simulink model "DEEE_centre_tri"  (R2026a)
settings: Solver=VariableStepDiscrete  StopTime=T_sim
values from neighbouring files (symbols this model uses):
  dt = 0.25    [params_DEEE.m]
  MTBF = 120    [params_DEEE.m]
  MTBF_B1 = 80    [params_DEEE.m]    (also in scenarios_DEEE.m = MTBF_B1_scenarios(i))
  MTBF_B2 = 120    [params_DEEE.m]
  MTBF_Mag = 200    [params_DEEE.m]
  MTBF_Opt = 60    [params_DEEE.m]
  MTTR = 4    [params_DEEE.m]
  MTTR_B1 = 6    [params_DEEE.m]
  MTTR_B2 = 4    [params_DEEE.m]
  MTTR_Mag = 3    [params_DEEE.m]
  MTTR_Opt = 2    [params_DEEE.m]
  tau_capt_GEM = 0.94    [params_DEEE.m]
undefined symbols (not defined in the file or in its folder): m, n
(part 1 of 2)
settings Model: Creator=fabri  LastModifiedBy=fabri

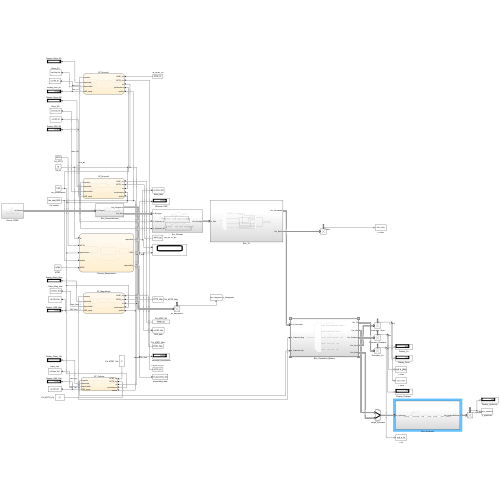
[thumbnail: Simulink's stored preview of the top-level diagram]
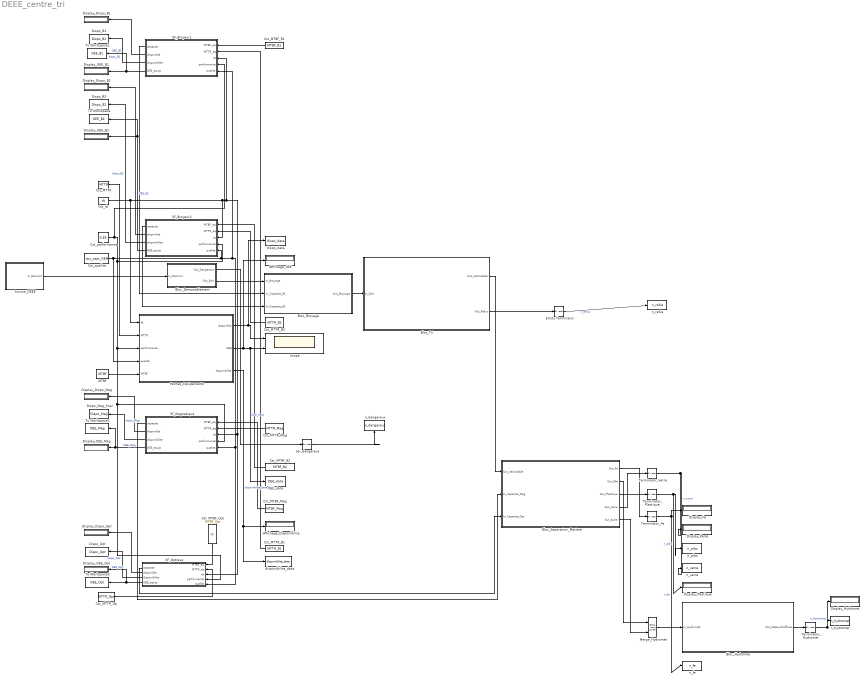
== system DEEE_centre_tri ==
  Affichage_Disponibilite : Display
  Affichage_OEE : Display
  Bloc_Broyage : Subsystem
  Bloc_Demantèlement : Subsystem
  Bloc_Hydromet : Subsystem
  Bloc_Separation_Matiere : Subsystem
  Bloc_Tri : Subsystem
  Cst_MTBF_B1 : Constant  Value=MTBF_B1
  Cst_MTBF_B2 : Constant  Value=MTBF_B2
  Cst_MTBF_Mag : Constant  Value=MTBF_Mag
  Cst_MTBF_Opt : Constant  Value=MTBF_Opt
  Cst_MTTR : Constant  Value=MTTR
  Cst_MTTR_B1 : Constant  Value=MTTR_B1
  Cst_MTTR_B2 : Constant  Value=MTTR_B2
  Cst_MTTR_Mag : Constant  Value=MTTR_Mag
  Cst_MTTR_Op : Constant  Value=MTTR_Opt
  Cst_dt : Constant  Value=dt
  Cst_performance : Constant  Value=0.85
  Cst_qualite : Constant  Value=tau_capt_GEM
  Display_Dispo_B1 : Display
  Display_Dispo_B2 : Display
  Display_Dispo_Mag : Display
  Display_Dispo_Opt : Display
  Display_Fe : Display
  Display_Hydromet : Display
  Display_OEE_B1 : Display
  Display_OEE_B2 : Display
  Display_OEE_Mag : Display
  Display_OEE_Opt : Display
  Display_Perre : Display
  Display_Plastique : Display
  Dispo_B1 : ToWorkspace  VariableName=Dispo_B1  SaveFormat=Timeseries  SampleTime=-1
  Dispo_B2 : ToWorkspace  VariableName=Dispo_B2  SaveFormat=Timeseries  SampleTime=-1
  Dispo_Mag_final : ToWorkspace  VariableName=Dispo_Mag  SaveFormat=Timeseries  SampleTime=-1
  Dispo_Opt : ToWorkspace  VariableName=Dispo_Opt  SaveFormat=Timeseries  SampleTime=-1
  Entity Terminator : EntityTerminator  InputPortMessageModes=m  NumberEntitiesArrived=on
      settings: OutputPortMap=o0
  MTBF : Constant  Value=MTBF
  Merge_Hydromet : EntityInputSwitch  InputPortMessageModes=m,m  OutputPortMessageModes=m
  OEE_data : ToWorkspace  VariableName=OEE_data  SaveFormat=Timeseries  SampleTime=-1
  Pannes_Equipements : Stateflow chart  TreatAsAtomicUnit=on
  SF_Broyeur1 : Stateflow chart  TreatAsAtomicUnit=on
  SF_Broyeur2 : Stateflow chart  TreatAsAtomicUnit=on
  SF_Magnetique : Stateflow chart  TreatAsAtomicUnit=on
  SF_Optique : Stateflow chart  TreatAsAtomicUnit=on
  Scope : Scope  NumInputPorts=2
      settings: ActiveDisplayYMinimum=-0.22946896582031268  ActiveDisplayYMaximum=1.3658829873046878
  Source_DEEE : Subsystem
  Terminator_Fe : EntityTerminator  InputPortMessageModes=m  NumberEntitiesArrived=on
      settings: OutputPortMap=o0
  Terminator_Hydromet : EntityTerminator  InputPortMessageModes=m  NumberEntitiesArrived=on
      settings: OutputPortMap=o0
  Terminator_Plastique : EntityTerminator  InputPortMessageModes=m  NumberEntitiesArrived=on
      settings: OutputPortMap=o0
  Terminator_Verre : EntityTerminator  InputPortMessageModes=m  NumberEntitiesArrived=on
      settings: OutputPortMap=o0
  To Workspace : ToWorkspace  VariableName=OEE_B2  SaveFormat=Timeseries  SampleTime=-1
  To Workspace1 : ToWorkspace  VariableName=OEE_B1  SaveFormat=Timeseries  SampleTime=-1
  To Workspace2 : ToWorkspace  VariableName=OEE_Mag  SaveFormat=Timeseries  SampleTime=-1
  To Workspace3 : ToWorkspace  VariableName=OEE_Opt  SaveFormat=Timeseries  SampleTime=-1
  dispo_data : ToWorkspace  VariableName=dispo_data  SaveFormat=Timeseries  SampleTime=-1
  disponibilite_data : ToWorkspace  VariableName=disponibilite_data  SaveFormat=Timeseries  SampleTime=-1
      settings: Save2DSignal=2-D array (concatenate along first dimension)
  n_dangereux : ToWorkspace  VariableName=n_dangereux  SaveFormat=Timeseries  SampleTime=-1
  n_fe : ToWorkspace  VariableName=n_fe  SaveFormat=Timeseries  SampleTime=-1
      settings: Save2DSignal=2-D array (concatenate along first dimension)
  n_hydromet : ToWorkspace  VariableName=n_hydromet  SaveFormat=Timeseries  SampleTime=-1
  n_plas : ToWorkspace  VariableName=n_plas  SaveFormat=Timeseries  SampleTime=-1
      settings: Save2DSignal=2-D array (concatenate along first dimension)
  n_refus : ToWorkspace  VariableName=n_refus  SaveFormat=Timeseries  SampleTime=-1
  n_verre : ToWorkspace  VariableName=n_verre  SaveFormat=Timeseries  SampleTime=-1
  ter_dangereux : EntityTerminator  InputPortMessageModes=m  NumberEntitiesArrived=on
      settings: OutputPortMap=o0
  wires:
  Source_DEEE/1(In_Demont) -> Bloc_Demantèlement/1(In_Demont)
  Cst_MTTR_Mag/1 -> SF_Magnetique/2(MTTR_eq)
  MTBF/1 -> Pannes_Equipements/5(MTBF)
  SF_Magnetique/3(disponibilite) -> Dispo_Mag_final/1  "dispo_Mag"
  Cst_qualite/1 -> SF_Magnetique/5(qualite), SF_Optique/5(qualite), SF_Broyeur1/5(qualite), SF_Broyeur2/5(qualite), Pannes_Equipements/4(qualite)
  Cst_performance/1 -> SF_Optique/4(performance), SF_Magnetique/4(performance), Pannes_Equipements/3(performance), SF_Broyeur2/4(performance), SF_Broyeur1/4(performance)
  Cst_dt/1 -> SF_Magnetique/3(dt), SF_Optique/3(dt), SF_Broyeur1/3(dt), SF_Broyeur2/3(dt), Pannes_Equipements/1(dt)
  Cst_MTTR/1 -> Pannes_Equipements/2(MTTR)
  Cst_MTBF_Opt/1 -> SF_Optique/1(MTBF_eq)
  Cst_MTBF_Mag/1 -> SF_Magnetique/1(MTBF_eq)
  Cst_MTTR_Op/1 -> SF_Optique/2(MTTR_eq)
  Cst_MTTR_B1/1 -> SF_Broyeur1/2(MTTR_eq)
  Cst_MTBF_B1/1 -> SF_Broyeur1/1(MTBF_eq)
  SF_Broyeur1/4(OEE_equip) -> To Workspace1/1, Display_OEE_B1/1  "OEE_B1"
  SF_Broyeur1/3(disponibilite) -> Dispo_B1/1  "dispo_B1"
  Pannes_Equipements/1(disponible) -> Scope/1, dispo_data/1
  SF_Broyeur1/2(disponible) -> Display_Dispo_B1/1
  SF_Broyeur1/1(capacite) -> Bloc_Broyage/2(In_Capacite_B1)
  SF_Broyeur2/4(OEE_equip) -> To Workspace/1, Display_OEE_B2/1  "OEE_B2"
  Cst_MTTR_B2/1 -> SF_Broyeur2/2(MTTR_eq)
  SF_Broyeur2/3(disponibilite) -> Dispo_B2/1  "dispo_B2"
  SF_Broyeur2/2(disponible) -> Display_Dispo_B2/1
  SF_Broyeur2/1(capacite) -> Bloc_Broyage/3(In_Capacite_B2)
  SF_Magnetique/4(OEE_equip) -> To Workspace2/1, Display_OEE_Mag/1  "OEE_Mag"
  Terminator_Fe/1 -> Display_Fe/1, n_fe/1  "n_fe"
  SF_Magnetique/2(disponible) -> Display_Dispo_Mag/1
  Cst_MTBF_B2/1 -> SF_Broyeur2/1(MTBF_eq)
  SF_Magnetique/1(capacite) -> Bloc_Separation_Matiere/2(In_Capacite_Mag)
  SF_Optique/4(OEE_equip) -> To Workspace3/1, Display_OEE_Opt/1  "OEE_Opt"
  SF_Optique/3(disponibilite) -> Dispo_Opt/1  "dispo_Opt"
  Bloc_Separation_Matiere/2(Out_Nfe) -> Merge_Hydromet/1
  SF_Optique/2(disponible) -> Display_Dispo_Opt/1
  Terminator_Hydromet/1 -> n_hydromet/1, Display_Hydromet/1  "n_hydromet"
  SF_Optique/1(capacite) -> Bloc_Separation_Matiere/3(In_Capacite_Opt)
  Pannes_Equipements/2(OEE) -> OEE_data/1, Scope/2, Affichage_OEE/1  "OEE_data"
  Bloc_Demantèlement/1(Out_Dangereux) -> ter_dangereux/1
  Bloc_Demantèlement/2(Out_Sain) -> Bloc_Broyage/1(In_Broyage)
  Pannes_Equipements/3(disponibilite) -> Affichage_Disponibilite/1, disponibilite_data/1  "disponibilite_data"
  Bloc_Broyage/1(Out_Broyage) -> Bloc_Tri/1(In_Sain)
  ter_dangereux/1 -> n_dangereux/1
  Bloc_Tri/1(Out_Valorisable) -> Bloc_Separation_Matiere/1(Out_Valorisable)
  Bloc_Tri/2(Out_Refus) -> Entity Terminator/1
  Entity Terminator/1 -> n_refus/1  "n_refus"
  Bloc_Separation_Matiere/5(Out_Autre) -> Merge_Hydromet/2
  Bloc_Separation_Matiere/1(Out_Fe) -> Terminator_Fe/1
  Bloc_Separation_Matiere/3(Out_Plastique) -> Terminator_Plastique/1
  Bloc_Hydromet/1(Out_MetauxRaffines) -> Terminator_Hydromet/1
  Bloc_Separation_Matiere/4(Out_Verre) -> Terminator_Verre/1
  Terminator_Verre/1 -> n_verre/1, Display_Perre/1  "n_verre"
  Terminator_Plastique/1 -> n_plas/1, Display_Plastique/1  "n_plas"
  Merge_Hydromet/1 -> Bloc_Hydromet/1(In_Hydromet)

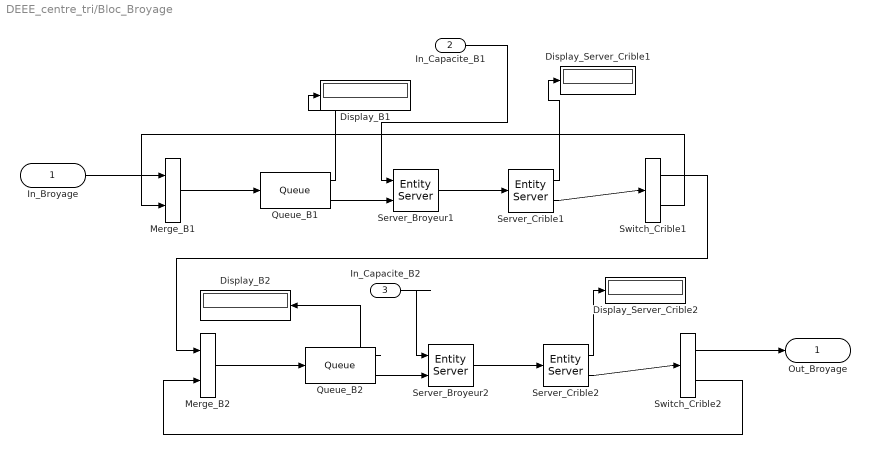
== system DEEE_centre_tri/Bloc_Broyage ==
  In_Broyage : Inport
  In_Capacite_B1 : Inport  Port=2
  In_Capacite_B2 : Inport  Port=3
  Display_B1 : Display
  Display_B2 : Display
  Display_Server_Crible1 : Display
  Display_Server_Crible2 : Display
  Merge_B1 : EntityInputSwitch  InputPortMessageModes=m,m  OutputPortMessageModes=m  SwitchingCriterion=Equiprobable
  Merge_B2 : EntityInputSwitch  InputPortMessageModes=m,m  OutputPortMessageModes=m  SwitchingCriterion=Equiprobable
  Queue_B1 : Queue  InputPortMessageModes=m  OutputPortMessageModes=n,m  Capacity=inf  NumberEntitiesInBlock=on
      settings: OutputPortMap=o1,o5
  Queue_B2 : Queue  InputPortMessageModes=m  OutputPortMessageModes=n,m  Capacity=inf  NumberEntitiesInBlock=on
      settings: OutputPortMap=o1,o5
  Server_Broyeur1 : EntityServer  InputPortMessageModes=n,m  OutputPortMessageModes=m  Capacity=10  ServiceTimeSource=Signal port  ServiceTimeAttributeName=tps_service  EntryAction=|
      | % =SÉCURITÉ DES ATTRIBUTS=
      | entity.grain_route       = 1;
      | entity.route_depollution = 2;
      | entity.valorisable       = 1;
      | cat = entity.categorie;
      | if isempty(cat) || ~isscalar(cat) || cat < 1 || cat > 4
      |     cat = 1;
      |     entity.categorie = 1;
      | end
      | 
      | % =BROYAGE PRIMAIRE (marteaux)=
      | r1_moy = [6.0, 7.0, 5.0, 8.0];
      | r1 = r1_moy(cat) * (1 + 0.15*(2*rand()-1));
      | r1 = max(r1, 1.0);
      | 
      | % Granulométrie d'entrée
      | if entity.granulometrie <= 0
      |     d50_init = [200, 100, 150, 120];
      |     entity.granulometrie = d50_init(cat) * (1 + 0.2*(2*rand()-1));
      | end
      | entity.granulometrie = entity.granulometrie / r1;
      | entity.granulometrie = max(entity.granulometrie, 0.5);
      | 
      | % Compteur de passages
      | entity.nb_passages = entity.nb_passages + 1;
      | 
      | % Temps de service
      | entity.tps_service = max(entity.masse / 6.0, 0.001);
      | 
      | % Rendement matière
      | entity.masse = max(entity.masse * 0.95, 0.0001);
      | % Énergie broyage primaire
      | energie_spec_B1 = 15.0;   % kWh/tonne
      | entity.energie_broyage = entity.energie_broyage + ...
      |     entity.masse * 1000 * energie_spec_B1 / 1000;  % kWh
      settings: InputPortMap=u0,u2
  Server_Broyeur2 : EntityServer  InputPortMessageModes=n,m  OutputPortMessageModes=m  Capacity=10  ServiceTimeSource=Signal port  ServiceTimeAttributeName=tps_service  EntryAction=|
      | % = SÉCURITÉ ATTRIBUTS =
      | entity.grain_route       = 1;
      | entity.route_depollution = 2;
      | entity.valorisable       = 1;
      | cat = entity.categorie;
      | if isempty(cat) || ~isscalar(cat) || cat < 1 || cat > 4
      |     cat = 1;
      |     entity.categorie = 1;
      | end
      | 
      | % = BROYAGE SECONDAIRE (boulets) =
      | r2_moy = [8.0, 10.0, 7.0, 9.0];
      | r2 = r2_moy(cat) * (1 + 0.15*(2*rand()-1));
      | r2 = max(r2, 1.0);
      | 
      | entity.granulometrie = entity.granulometrie / r2;
      | entity.granulometrie = max(entity.granulometrie, 0.1);
      | 
      | % Compteur de passages
      | entity.nb_passages = entity.nb_passages + 1;
      | 
      | % Temps de service
      | entity.tps_service = max(entity.masse / 3.0, 0.001);
      | 
      | % Rendement matière
      | entity.masse = max(entity.masse * 0.97, 0.0001);
      | % Énergie broyage secondaire
      | energie_spec_B2 = 25.0;   % kWh/tonne
      | entity.energie_broyage = entity.energie_broyage + ...
      |     entity.masse * 1000 * energie_spec_B2 / 1000;
      | 
      | % Énergie cribles + convoyeurs
      | energie_spec_conv = 2.0;   % kWh/tonne
      | entity.energie_broyage = entity.energie_broyage + ...
      |     entity.masse * 1000 * energie_spec_conv / 1000;
      settings: InputPortMap=u0,u2
  Server_Crible1 : EntityServer  InputPortMessageModes=m  OutputPortMessageModes=n,m  Capacity=10  ServiceTimeSource=Attribute  ServiceTimeAttributeName=tps_service  EntryAction=|  NumberEntitiesDeparted=on
      | % = SÉCURITÉ ATTRIBUTS =
      | entity.route_depollution = 2;
      | entity.valorisable       = 1;
      | if ~isscalar(entity.categorie) || entity.categorie < 1 || entity.categorie > 4
      |     entity.categorie = 1;
      | end
      | 
      | % = CRIBLAGE 1 — seuil 10mm =
      | entity.tps_service = 0.005;
      | entity.grain_route = 1;  % passant par défaut
      | 
      | if entity.nb_passages >= 3
      |     entity.grain_route = 1;  % forcer sortie après 3 passages
      | elseif entity.granulometrie > 10.0
      |     entity.grain_route = 2;  % refus → recirculation B1
      | end
      settings: OutputPortMap=o0,o9
  Server_Crible2 : EntityServer  InputPortMessageModes=m  OutputPortMessageModes=n,m  Capacity=10  ServiceTimeSource=Attribute  ServiceTimeAttributeName=tps_service  EntryAction=|  NumberEntitiesDeparted=on
      | % = SÉCURITÉ ATTRIBUTS =
      | entity.route_depollution = 2;
      | entity.valorisable       = 1;
      | if ~isscalar(entity.categorie) || entity.categorie < 1 || entity.categorie > 4
      |     entity.categorie = 1;
      | end
      | 
      | % = CRIBLAGE 2 — seuil 2mm =
      | entity.tps_service = 0.005;
      | entity.grain_route = 1;  % passant par défaut
      | 
      | if entity.nb_passages >= 6
      |     entity.grain_route = 1;  % forcer la sortie après 6 passages total
      | elseif entity.granulometrie > 2.0
      |     entity.grain_route = 2;  % refus → recirculation B2
      | end
      settings: OutputPortMap=o0,o9
  Switch_Crible1 : EntityOutputSwitch  InputPortMessageModes=m  OutputPortMessageModes=m,m  SwitchingCriterion=From attribute  SwitchAttributeName=grain_route
  Switch_Crible2 : EntityOutputSwitch  InputPortMessageModes=m  OutputPortMessageModes=m,m  SwitchingCriterion=From attribute  SwitchAttributeName=grain_route
  Out_Broyage : Outport
  wires:
  Server_Crible2/2 -> Switch_Crible2/1
  Server_Crible1/2 -> Switch_Crible1/1
  Server_Broyeur2/1 -> Server_Crible2/1
  Server_Broyeur1/1 -> Server_Crible1/1
  Queue_B2/2 -> Server_Broyeur2/2
  Queue_B1/2 -> Server_Broyeur1/2
  Merge_B1/1 -> Queue_B1/1
  Merge_B2/1 -> Queue_B2/1
  Switch_Crible1/1 -> Merge_B2/1
  Switch_Crible1/2 -> Merge_B1/2
  Switch_Crible2/2 -> Merge_B2/2
  Switch_Crible2/1 -> Out_Broyage/1
  Queue_B1/1 -> Display_B1/1
  Queue_B2/1 -> Display_B2/1
  Server_Crible2/1 -> Display_Server_Crible2/1
  Server_Crible1/1 -> Display_Server_Crible1/1
  In_Broyage/1 -> Merge_B1/1
  In_Capacite_B1/1 -> Server_Broyeur1/1
  In_Capacite_B2/1 -> Server_Broyeur2/1

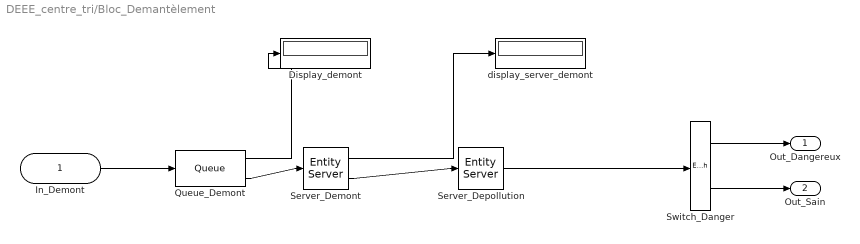
== system DEEE_centre_tri/Bloc_Demantèlement ==
  In_Demont : Inport
  Display_demont : Display
  Queue_Demont : Queue  InputPortMessageModes=m  OutputPortMessageModes=n,m  NumberEntitiesDeparted=on
      settings: OutputPortMap=o0,o5
  Server_Demont : EntityServer  InputPortMessageModes=m  OutputPortMessageModes=n,m  Capacity=20  EntryAction=|  NumberEntitiesInBlock=on
      | % Temps de démantèlement par catégorie [h]
      | % GEM=45min  PAM=15min  ECR=20min  IT=30min
      | t_demont = [0.0375, 0.0125, 0.0165, 0.0250];
      | cat = entity.categorie;
      | entity.tps_service = t_demont(cat)
      | 
      | % Granulométrie des composants après démantèlement [mm]
      | % Moyenne pondérée par composition matière
      | d50_metaux    = [150, 100,  80, 100];
      | d50_plastique = [300, 200, 250, 180];
      | d50_cartes    = [ 80,  60, 120, 150];
      | 
      | entity.granulometrie = ...
      |     (entity.masse_fe + entity.masse_nfe) / entity.masse * d50_metaux(cat) + ...
      |     entity.masse_plastique / entity.masse * d50_plastique(cat) + ...
      |     entity.masse_autre / entity.masse * d50_cartes(cat) + ...
      |     entity.masse_verre / entity.masse * 50;
      | 
      | % Variabilité ±20%
      | entity.granulometrie = entity.granulometrie * (1 + 0.20*(2*rand()-1));
      | entity.granulometrie = max(entity.granulometrie, 5);
      settings: OutputPortMap=o1,o9
  Server_Depollution : EntityServer  InputPortMessageModes=m  OutputPortMessageModes=m  Capacity=20  EntryAction=|
      | % Probabilité des substances dangereuses par catégorie
      | % GEM=15%  PAM=8%  ECR=20%  IT=12%
      | p_danger = [0.15, 0.08, 0.20, 0.12];
      | cat = entity.categorie;
      | 
      | % Détection substances dangereuses
      | if rand() < p_danger(cat)
      |     entity.dangereux = 1;
      | else
      |     entity.dangereux = 0;
      | end
      | 
      | % Masse batteries par catégorie [kg]
      | m_bat = [0.5, 0.1, 0.3, 0.2];
      | if entity.dangereux == 1
      |     entity.masse_bat = entity.masse * 1000 * m_bat(cat) / 35;
      |     entity.masse_Hg  = entity.masse * 1000 * 0.005;
      | else
      |     entity.masse_bat = 0;
      |     entity.masse_Hg  = 0;
      | end
      | 
      | % Mise à jour masse après extraction dangereuses
      | entity.masse = entity.masse - entity.masse_bat/1000;
      | entity.masse = max(entity.masse, 0.001);
      | 
      | % Temps de dépollution
      | entity.tps_service = 0.005;  % 18 secondes
      | 
      | % Routage CORRIGÉ
      | % Out_Dangereux = port 1, Out_Sain = port 2
      | if entity.dangereux == 1
      |     entity.route_depollution = 1;  % port 1 → Out_Dangereux
      | else
      |     entity.route_depollution = 2;  % port 2 → Out_Sain
      | end
  Switch_Danger : EntityOutputSwitch  InputPortMessageModes=m  OutputPortMessageModes=m,m  SwitchingCriterion=From attribute  SwitchAttributeName=route_depollution
  display_server_demont : Display
  Out_Dangereux : Outport
  Out_Sain : Outport  Port=2
  wires:
  In_Demont/1 -> Queue_Demont/1
  Queue_Demont/2 -> Server_Demont/1
  Server_Demont/2 -> Server_Depollution/1
  Server_Depollution/1 -> Switch_Danger/1
  Queue_Demont/1 -> Display_demont/1
  Server_Demont/1 -> display_server_demont/1
  Switch_Danger/2 -> Out_Sain/1
  Switch_Danger/1 -> Out_Dangereux/1

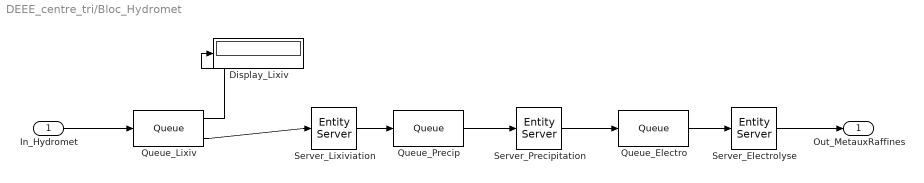
== system DEEE_centre_tri/Bloc_Hydromet ==
  In_Hydromet : Inport
  Display_Lixiv : Display
  Queue_Electro : Queue  InputPortMessageModes=m  OutputPortMessageModes=m
  Queue_Lixiv : Queue  InputPortMessageModes=m  OutputPortMessageModes=n,m  NumberEntitiesInBlock=on
      settings: OutputPortMap=o1,o5
  Queue_Precip : Queue  InputPortMessageModes=m  OutputPortMessageModes=m
  Server_Electrolyse : EntityServer  InputPortMessageModes=m  OutputPortMessageModes=m  Capacity=1  EntryAction=|
      | % Électrolyse—raffinage final
      | % Électrolyse Cu : anode impure → cathode pure 99.99%
      | % Coupellation Au/Ag : fusion + oxydation impuretés
      | 
      | % Rendements électrolyse
      | eta_electro_Cu = 0.99;
      | eta_electro_Au = 0.998;
      | eta_electro_Ag = 0.995;
      | 
      | % Masses finales raffinées [kg/g]
      | entity.masse_Cu = entity.masse_Cu * eta_electro_Cu;
      | entity.masse_Au = entity.masse_Au * eta_electro_Au;
      | entity.masse_Ag = entity.masse_Ag * eta_electro_Ag;
      | 
      | % Valeur finale après raffinage complet
      | entity.valeur_euro = entity.masse_Cu * 8.5 + ...
      |     entity.masse_Au  * 60.0 + ...
      |     entity.masse_Ag  * 0.8;
      | 
      | % Temps électrolyse—plus long pour Cu
      | % [GEM, PAM, ECR, IT]
      | t_electro = [0.15, 0.10, 0.20, 0.25];
      | cat = entity.categorie;
      | entity.tps_service = t_electro(cat);
      | % Calcul rendements globaux hydromet
      | if entity.masse_Cu_init > 0
      |     entity.rendement_Cu = entity.masse_Cu / entity.masse_Cu_init * 100;
      | else
      |     entity.rendement_Cu = 0;
      | end
      | if entity.masse_Au_init > 0
      |     entity.rendement_Au = entity.masse_Au / entity.masse_Au_init * 100;
      | else
      |     entity.rendement_Au = 0;
      | end
      | if entity.masse_Ag_init > 0
      |     entity.rendement_Ag = entity.masse_Ag / entity.masse_Ag_init * 100;
      | else
      |     entity.rendement_Ag = 0;
      | end
      | 
      | % Valeur économique finale
      | entity.valeur_euro = entity.masse_Cu * 8.5 + ...
      |     entity.masse_Au  * 60.0 + ...
      |     entity.masse_Ag  * 0.8;
      | % --- ÉNERGIE ÉLECTROLYSE ---
      | % Cu : 0.35 kWh/kg Cu récupéré
      | % Au/Ag : 0.05 kWh/g métal précieux
      | energie_Cu    = entity.masse_Cu * 1000 * 0.35;
      | energie_AuAg  = (entity.masse_Au + entity.masse_Ag) * 0.05;
      | entity.energie_electro = energie_Cu + energie_AuAg;
      | 
      | % --- ÉNERGIE TOTALE HYDROMET ---
      | entity.energie_totale = entity.energie_lixiv + ...
      |     entity.energie_precip + ...
      |     entity.energie_electro;
      | 
      | % --- EFFLUENTS FINAUX ---
      | % Traitement final — neutralisation à la chaux
      | entity.pH_effluent = 7.0 + randn() * 0.3;  % pH ≈ 7 après traitement
      | entity.conc_acide  = 0;  % acide neutralisé
      | % Énergie totale process complet
      | entity.energie_totale_process = entity.energie_broyage + ...
      |     entity.energie_tri + ...
      |     entity.energie_separation + ...
      |     entity.energie_lixiv + ...
      |     entity.energie_precip + ...
      |     entity.energie_electro;
      | %% === RÉCUPÉRATION CHALEUR ÉLECTROLYSE ===
      | 
      | % Chaleur effet Joule — 30% de l'énergie électrique dissipée
      | facteur_joule    = 0.30;
      | Q_joule_kWh      = entity.energie_electro * facteur_joule;
      | 
      | % Récupération via échangeur sur l'électrolyte chaud
      | eta_recup_electro = 0.65;   % rendement récupération électrolyse
      | Q_recup_electro   = eta_recup_electro * Q_joule_kWh;
      | 
      | % Mise à jour chaleur récupérée totale
      | entity.chaleur_recuperee = entity.chaleur_recuperee + Q_recup_electro;
      | 
      | % Énergie électrolyse nette
      | entity.energie_electro = entity.energie_electro - Q_recup_electro;
      | entity.energie_electro = max(entity.energie_electro, 0);
      | 
      | % Taux de récupération global [%]
      | energie_brute_totale = entity.energie_broyage + entity.energie_tri + ...
      |     entity.energie_separation + entity.energie_lixiv + ...
      |     entity.energie_precip + entity.energie_electro + ...
      |     entity.chaleur_recuperee;
      | 
      | if energie_brute_totale > 0
      |     entity.taux_recuperation = entity.chaleur_recuperee / ...
      |         energie_brute_totale * 100;
      | end
      | 
      | % Énergie totale nette finale
      | entity.energie_totale_process = entity.energie_broyage + ...
      |     entity.energie_tri + ...
      |     entity.energie_separation + ...
      |     entity.energie_lixiv_nette + ...
      |     entity.energie_precip + ...
      |     entity.energie_electro;
  Server_Lixiviation : EntityServer  InputPortMessageModes=m  OutputPortMessageModes=m  Capacity=1  EntryAction=|
      | %% === LIXIVIATION AVEC THERMIQUE + ENERGIE + EFFLUENTS ===
      | 
      | % --- 1. MODÉLISATION THERMIQUE ---
      | % Température initiale cuve [°C]
      | T_amb     = 20.0;   % température ambiante
      | T_cible   = 70.0;   % température opératoire cible
      | tau_chauf = 2.0;    % constante de temps chauffage [h]
      | 
      | % Montée en température (modèle du premier ordre)
      | % T(t) = T_cible - (T_cible - T_amb) * exp(-t/tau)
      | % On utilise tps_service comme proxy du temps
      | t_lixiv_base = 0.025;
      | entity.tps_service = t_lixiv_base * (entity.granulometrie / 2.0)^0.3;
      | entity.tps_service = max(entity.tps_service, 0.005);
      | entity.tps_service = min(entity.tps_service, 0.10);
      | 
      | % Température atteinte en fin de lixiviation
      | entity.temp_cuve = T_cible - (T_cible - T_amb) * ...
      |     exp(-entity.tps_service / tau_chauf);
      | 
      | % --- 2. RENDEMENTS CORRIGÉS PAR TEMPÉRATURE ---
      | % η(T) = η_ref × (1 + α × (T - T_ref))
      | T_ref  = 60.0;   % température de référence [°C]
      | alpha  = 0.005;  % coefficient température [1/°C]
      | facteur_T = 1 + alpha * (entity.temp_cuve - T_ref);
      | facteur_T = max(0.8, min(1.2, facteur_T));  % limité ±20%
      | 
      | cat = entity.categorie;
      | eta_lixiv_Cu = [0.88, 0.90, 0.85, 0.92];
      | eta_lixiv_Au = [0.80, 0.82, 0.85, 0.87];
      | eta_lixiv_Ag = [0.83, 0.85, 0.88, 0.90];
      | 
      | % Application correction thermique
      | entity.eta_lixiv_reel = eta_lixiv_Cu(cat) * facteur_T;
      | entity.masse_Cu = entity.masse_Cu * entity.eta_lixiv_reel;
      | entity.masse_Au = entity.masse_Au * eta_lixiv_Au(cat) * facteur_T;
      | entity.masse_Ag = entity.masse_Ag * eta_lixiv_Ag(cat) * facteur_T;
      | 
      | % --- 3. BILAN ÉNERGÉTIQUE LIXIVIATION ---
      | % Énergie chauffage : Q = m_cuve × Cp × ΔT / η_chauffage
      | % Simplifié : 0.8 kWh/kg de matière traitée
      | energie_spec_lixiv = 0.8;   % kWh/kg
      | entity.energie_lixiv = entity.masse * 1000 * energie_spec_lixiv;
      | 
      | % --- 4. EFFLUENTS ACIDES ---
      | % Volume effluent = 4 L/kg traité (moyenne industrielle)
      | vol_spec = [3.5, 4.0, 4.5, 5.0];   % L/kg par catégorie
      | entity.volume_effluent = entity.masse * 1000 * vol_spec(cat);
      | 
      | % pH effluent en sortie lixiviation
      | % Plus la teneur en métaux est élevée, plus le pH remonte
      | pH_base = 1.2;
      | entity.pH_effluent = pH_base + 0.5 * entity.eta_lixiv_reel;
      | 
      | % Concentration acide résiduel [mol/L]
      | entity.conc_acide = 0.5 * (1 - entity.eta_lixiv_reel);
      | %% === MODULE RÉCUPÉRATION DE CHALEUR ===
      | 
      | % Paramètres échangeur de chaleur
      | eta_echangeur = 0.75;   % rendement échangeur à plaques
      | Cp_eau        = 4.18;   % kJ/kg·°C
      | T_effluent    = entity.temp_cuve;   % température effluent sortant
      | T_reseau      = 20.0;   % température eau réseau entrant [°C]
      | T_prechauffee = T_reseau + eta_echangeur * (T_effluent - T_reseau);
      | 
      | % Masse effluent [kg] = volume [L] × densité ≈ 1 kg/L
      | masse_effluent = entity.volume_effluent;   % kg
      | 
      | % Chaleur récupérée [kWh]
      | % Q = m × Cp × ΔT / 3600 (conversion kJ → kWh)
      | Q_recuperee = masse_effluent * Cp_eau * ...
      |     (T_effluent - T_reseau) * eta_echangeur / 3600;
      | entity.chaleur_recuperee = Q_recuperee;
      | 
      | % Chaleur nécessaire SANS récupération [kWh]
      | % Q_brute = m × Cp × (T_cible - T_reseau) / 3600
      | Q_brute = masse_effluent * Cp_eau * ...
      |     (entity.temp_cuve - T_reseau) / 3600;
      | 
      | % Énergie lixiviation nette AVEC récupération
      | entity.energie_lixiv_nette = max(entity.energie_lixiv - Q_recuperee, 0);
      | 
      | % Taux de récupération [%]
      | if Q_brute > 0
      |     entity.taux_recuperation = Q_recuperee / Q_brute * 100;
      | else
      |     entity.taux_recuperation = 0;
      | end
      | 
      | % Mise à jour énergie totale avec récupération
      | entity.energie_totale_process = entity.energie_broyage + ...
      |     entity.energie_tri + ...
      |     entity.energie_separation + ...
      |     entity.energie_lixiv_nette + ...
      |     entity.energie_precip + ...
      |     entity.energie_electro;
  Server_Precipitation : EntityServer  InputPortMessageModes=m  OutputPortMessageModes=m  Capacity=1  EntryAction=|
      | % Précipitation sélective—séparation Cu/Au/Ag
      | % Étape 1 : ciment Cu (Fe + CuSO4 → FeSO4 + Cu)
      | % Étape 2 : NaOH pour précipiter Au/Ag
      | 
      | % Rendements précipitation
      | eta_precip_Cu = 0.95;
      | eta_precip_Au = 0.92;
      | eta_precip_Ag = 0.90;
      | 
      | % Masses après précipitation
      | entity.masse_Cu = entity.masse_Cu * eta_precip_Cu;
      | entity.masse_Au = entity.masse_Au * eta_precip_Au;
      | entity.masse_Ag = entity.masse_Ag * eta_precip_Ag;
      | 
      | % Temps précipitation—plus rapide que lixiviation
      | entity.tps_service = 0.075
      | 
      | % Mise à jour valeur après pertes précipitation
      | entity.valeur_euro = entity.masse_Cu * 8.5 + ...
      |     entity.masse_Au  * 60.0 + ...
      |     entity.masse_Ag  * 0.8;
      | % --- ÉNERGIE PRÉCIPITATION ---
      | energie_spec_precip = 0.1;   % kWh/kg
      | entity.energie_precip = entity.masse * 1000 * energie_spec_precip;
      | 
      | % --- EFFLUENTS PRÉCIPITATION ---
      | % Neutralisation partielle — pH remonte
      | entity.pH_effluent = entity.pH_effluent + 1.5;
      | entity.conc_acide  = entity.conc_acide * 0.3;  % 70% neutralisé
      | entity.volume_effluent = entity.volume_effluent * 0.8;  % évaporation
      | %% === RÉCUPÉRATION CHALEUR PRÉCIPITATION ===
      | 
      | % Chaleur de réaction exothermique [kWh]
      | % Cémentation Cu : ΔH ≈ -210 kJ/mol Cu
      | % Masse molaire Cu = 63.5 g/mol
      | moles_Cu = entity.masse_Cu * 1000 / 0.0635;   % moles Cu précipité
      | DH_cementation = 210;   % kJ/mol
      | Q_reaction_kJ  = moles_Cu * DH_cementation;
      | Q_reaction_kWh = Q_reaction_kJ / 3600;
      | 
      | % Récupération chaleur réaction
      | eta_recup_precip = 0.60;   % rendement récupération précipitation
      | Q_recup_precip   = eta_recup_precip * Q_reaction_kWh;
      | 
      | % Mise à jour énergie précipitation nette
      | entity.chaleur_recuperee  = entity.chaleur_recuperee + Q_recup_precip;
      | entity.energie_precip     = max(entity.energie_precip - Q_recup_precip, 0);
      | 
      | % Température effluent précipitation
      | entity.temp_cuve = 40.0 + randn() * 3.0;   % °C ≈ 40°C
  Out_MetauxRaffines : Outport
  wires:
  In_Hydromet/1 -> Queue_Lixiv/1
  Server_Precipitation/1 -> Queue_Electro/1
  Server_Lixiviation/1 -> Queue_Precip/1
  Queue_Precip/1 -> Server_Precipitation/1
  Queue_Electro/1 -> Server_Electrolyse/1
  Server_Electrolyse/1 -> Out_MetauxRaffines/1
  Queue_Lixiv/2 -> Server_Lixiviation/1
  Queue_Lixiv/1 -> Display_Lixiv/1

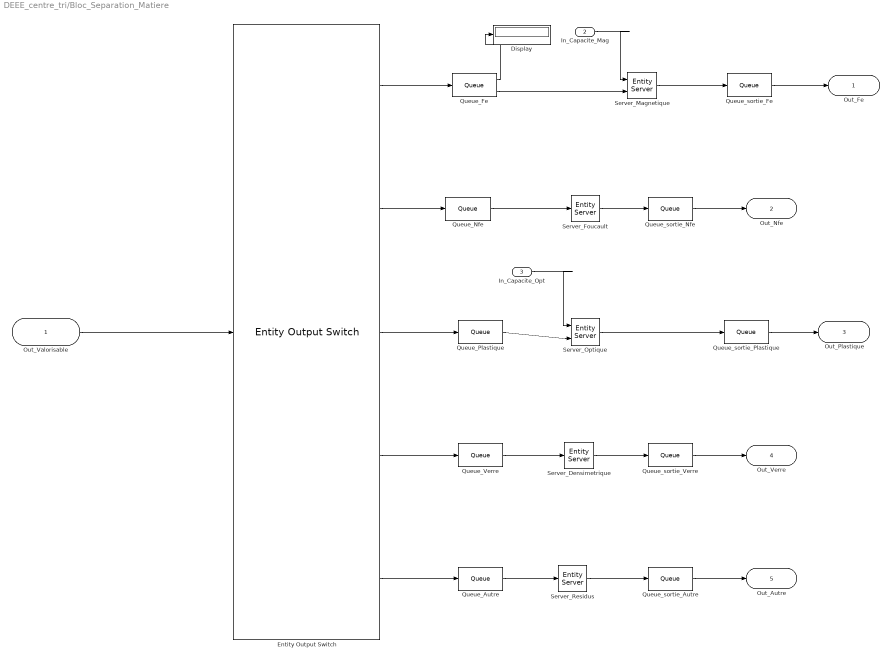
== system DEEE_centre_tri/Bloc_Separation_Matiere ==
  Out_Valorisable : Inport
  In_Capacite_Mag : Inport  Port=2
  In_Capacite_Opt : Inport  Port=3
  Display : Display
  Entity Output Switch : EntityOutputSwitch  InputPortMessageModes=m  OutputPortMessageModes=m,m,m,m,m  NumberOutputPorts=5  SwitchingCriterion=From attribute  SwitchAttributeName=fraction_dominante
      settings: OutputPortMap=o0,o1,o2,o3,o4
  Queue_Autre : Queue  InputPortMessageModes=m  OutputPortMessageModes=m
  Queue_Fe : Queue  InputPortMessageModes=m  OutputPortMessageModes=n,m  NumberEntitiesInBlock=on
      settings: OutputPortMap=o1,o5
  Queue_Nfe : Queue  InputPortMessageModes=m  OutputPortMessageModes=m
  Queue_Plastique : Queue  InputPortMessageModes=m  OutputPortMessageModes=m
  Queue_Verre : Queue  InputPortMessageModes=m  OutputPortMessageModes=m
  Queue_sortie_Autre : Queue  InputPortMessageModes=m  OutputPortMessageModes=m
  Queue_sortie_Fe : Queue  InputPortMessageModes=m  OutputPortMessageModes=m
  Queue_sortie_Nfe : Queue  InputPortMessageModes=m  OutputPortMessageModes=m
  Queue_sortie_Plastique : Queue  InputPortMessageModes=m  OutputPortMessageModes=m
  Queue_sortie_Verre : Queue  InputPortMessageModes=m  OutputPortMessageModes=m
  Server_Densimetrique : EntityServer  InputPortMessageModes=m  OutputPortMessageModes=m  Capacity=1  ServiceTimeSource=Attribute  ServiceTimeAttributeName=tps_service  EntryAction=|
      | % Rendements de séparation par procédé
      | % === SÉPARATION DENSIMÉTRIQUE — Verre ===
      | eta_densi = 0.80;
      | 
      | % Masse récupérée verre
      | entity.masse_recuperee = entity.masse_verre * eta_densi;
      | 
      | % Impuretés dans le produit verre
      | impurete_plas   = entity.masse_plastique * 0.02;
      | impurete_autre  = entity.masse_autre     * 0.02;
      | masse_sortie_Verre = entity.masse_recuperee + impurete_plas + impurete_autre;
      | 
      | % KPIs séparation densimétrique
      | if masse_sortie_Verre > 0
      |     entity.purete_Verre    = entity.masse_recuperee / masse_sortie_Verre;
      | else
      |     entity.purete_Verre    = 0;
      | end
      | entity.rendement_Verre = entity.masse_recuperee / max(entity.masse_verre, 0.0001);
      | entity.pertes_Verre    = entity.masse_verre - entity.masse_recuperee;
      | 
      | % Temps service
      | entity.tps_service = entity.masse / 2.0;
  Server_Foucault : EntityServer  InputPortMessageModes=m  OutputPortMessageModes=m  Capacity=1  ServiceTimeSource=Attribute  ServiceTimeAttributeName=tps_service  EntryAction=|
      | % Rendements de séparation par procédé
      | % === COURANTS DE FOUCAULT — Métaux non ferreux (Cu, Al) ===
      | eta_foucault = 0.85;
      | 
      | % Masse récupérée NFe
      | entity.masse_recuperee = entity.masse_nfe * eta_foucault;
      | 
      | % Impuretés dans le produit NFe
      | impurete_fe     = entity.masse_fe    * 0.02;
      | impurete_autre  = entity.masse_autre * 0.03;
      | masse_sortie_NFe = entity.masse_recuperee + impurete_fe + impurete_autre;
      | 
      | % KPIs courants de Foucault
      | if masse_sortie_NFe > 0
      |     entity.purete_NFe    = entity.masse_recuperee / masse_sortie_NFe;
      | else
      |     entity.purete_NFe    = 0;
      | end
      | entity.rendement_NFe = entity.masse_recuperee / max(entity.masse_nfe, 0.0001);
      | entity.pertes_NFe    = entity.masse_nfe - entity.masse_recuperee;
      | 
      | % Temps service
      | entity.tps_service = entity.masse / 4.0;
      | % Énergie courants de Foucault
      | energie_spec_nfe = 3.0;   % kWh/tonne
      | entity.energie_separation = entity.energie_separation + ...
      |     entity.masse * 1000 * energie_spec_nfe / 1000;
  Server_Magnetique : EntityServer  InputPortMessageModes=n,m  OutputPortMessageModes=m  Capacity=1  ServiceTimeSource=Signal port  ServiceTimeAttributeName=tps_service  EntryAction=|
      | % Rendements de séparation par procédé
      | % === SÉPARATEUR MAGNÉTIQUE — Métaux ferreux ===
      | eta_sep   = [0.95, 0.85, 0.92, 0.80, 0.70];
      | debit_sep = [6.0,  4.0,  4.0,  2.0,  3.0];
      | frac = entity.fraction_dominante;
      | 
      | % Temps de service
      | entity.tps_service = entity.masse / debit_sep(frac);
      | 
      | % Masse récupérée fraction cible (Fe)
      | entity.masse_recuperee = entity.masse_fe * eta_sep(frac);
      | 
      | % Impuretés dans le produit Fe (contamination NFe et autre)
      | impurete_nfe    = entity.masse_nfe    * 0.05;  % 5% NFe passe avec Fe
      | impurete_autre  = entity.masse_autre  * 0.02;  % 2% autre passe avec Fe
      | masse_sortie_Fe = entity.masse_recuperee + impurete_nfe + impurete_autre;
      | 
      | % KPIs séparateur magnétique
      | if masse_sortie_Fe > 0
      |     entity.purete_Fe    = entity.masse_recuperee / masse_sortie_Fe;
      | else
      |     entity.purete_Fe    = 0;
      | end
      | entity.rendement_Fe = entity.masse_recuperee / max(entity.masse_fe, 0.0001);
      | entity.pertes_Fe    = entity.masse_fe - entity.masse_recuperee;
      | % Énergie séparateur magnétique
      | energie_spec_mag = 1.0;   % kWh/tonne
      | entity.energie_separation = entity.energie_separation + ...
      |     entity.masse * 1000 * energie_spec_mag / 1000;
      settings: InputPortMap=u0,u2
  Server_Optique : EntityServer  InputPortMessageModes=n,m  OutputPortMessageModes=m  Capacity=1  ServiceTimeSource=Signal port  ServiceTimeAttributeName=tps_service  EntryAction=|
      | % Rendements de séparation par procédé
      | % === TRI OPTIQUE — Plastiques ===
      | eta_optique = 0.92;
      | 
      | % Masse récupérée plastiques
      | entity.masse_recuperee = entity.masse_plastique * eta_optique;
      | 
      | % Impuretés dans le produit plastique
      | impurete_verre  = entity.masse_verre  * 0.03;
      | impurete_autre  = entity.masse_autre  * 0.04;
      | masse_sortie_Plas = entity.masse_recuperee + impurete_verre + impurete_autre;
      | 
      | % KPIs tri optique
      | if masse_sortie_Plas > 0
      |     entity.purete_Plas    = entity.masse_recuperee / masse_sortie_Plas;
      | else
      |     entity.purete_Plas    = 0;
      | end
      | entity.rendement_Plas = entity.masse_recuperee / max(entity.masse_plastique, 0.0001);
      | entity.pertes_Plas    = entity.masse_plastique - entity.masse_recuperee;
      | 
      | % Temps service
      | entity.tps_service = entity.masse / 4.0;
      | % Énergie tri optique séparation
      | energie_spec_opt = 5.0;   % kWh/tonne
      | entity.energie_separation = entity.energie_separation + ...
      |     entity.masse * 1000 * energie_spec_opt / 1000;
      settings: InputPortMap=u0,u2
  Server_Residus : EntityServer  InputPortMessageModes=m  OutputPortMessageModes=m  Capacity=1  ServiceTimeSource=Attribute  ServiceTimeAttributeName=tps_service  EntryAction=|
      | % Rendements de séparation par procédé
      | % [Magnétique, Foucault, Optique, Densimétrique, Résidus]
      | eta_sep   = [0.95, 0.85, 0.92, 0.80, 0.70];
      | 
      | % Débits de traitement [t/h] par procédé
      | debit_sep = [6.0,  4.0,  4.0,  2.0,  3.0];
      | 
      | frac = entity.fraction_dominante;
      | 
      | % Temps de service selon débit du procédé
      | entity.tps_service     = entity.masse / debit_sep(frac);
      | 
      | % Masse récupérée après séparation
      | entity.masse_recuperee = entity.masse * eta_sep(frac);
  Out_Fe : Outport
  Out_Nfe : Outport  Port=2
  Out_Plastique : Outport  Port=3
  Out_Verre : Outport  Port=4
  Out_Autre : Outport  Port=5
  wires:
  Entity Output Switch/2 -> Queue_Nfe/1
  Queue_Verre/1 -> Server_Densimetrique/1
  Entity Output Switch/4 -> Queue_Verre/1
  Entity Output Switch/3 -> Queue_Plastique/1
  Queue_Nfe/1 -> Server_Foucault/1
  Entity Output Switch/1 -> Queue_Fe/1
  Out_Valorisable/1 -> Entity Output Switch/1
  Queue_Autre/1 -> Server_Residus/1
  Entity Output Switch/5 -> Queue_Autre/1
  Server_Foucault/1 -> Queue_sortie_Nfe/1
  Server_Optique/1 -> Queue_sortie_Plastique/1
  Server_Densimetrique/1 -> Queue_sortie_Verre/1
  Server_Residus/1 -> Queue_sortie_Autre/1
  Queue_sortie_Fe/1 -> Out_Fe/1
  Queue_sortie_Nfe/1 -> Out_Nfe/1
  Queue_sortie_Plastique/1 -> Out_Plastique/1
  Queue_sortie_Verre/1 -> Out_Verre/1
  Queue_sortie_Autre/1 -> Out_Autre/1
  Server_Magnetique/1 -> Queue_sortie_Fe/1
  Queue_Fe/2 -> Server_Magnetique/2
  Queue_Plastique/1 -> Server_Optique/2
  Queue_Fe/1 -> Display/1
  In_Capacite_Mag/1 -> Server_Magnetique/1
  In_Capacite_Opt/1 -> Server_Optique/1

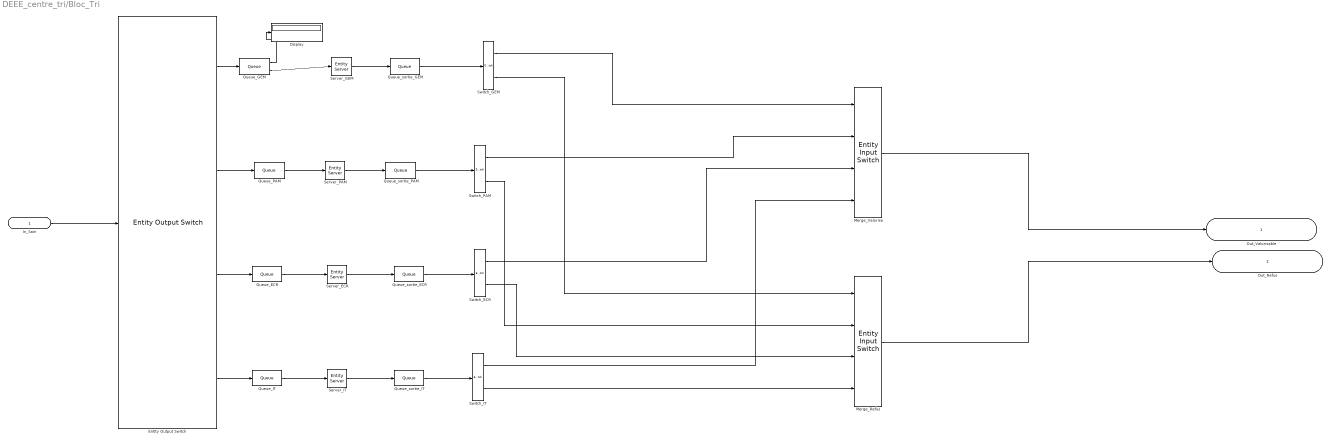
== system DEEE_centre_tri/Bloc_Tri ==
  In_Sain : Inport
  Display : Display
  Entity Output Switch : EntityOutputSwitch  InputPortMessageModes=m  OutputPortMessageModes=m,m,m,m  NumberOutputPorts=4  SwitchingCriterion=From attribute  SwitchAttributeName=categorie
      settings: OutputPortMap=o0,o1,o2,o3
  Merge_Refus : EntityInputSwitch  InputPortMessageModes=m,m,m,m  OutputPortMessageModes=m  NumberInputPorts=4
      settings: InputPortMap=u1,u2,u3,u4
  Merge_Valorise : EntityInputSwitch  InputPortMessageModes=m,m,m,m  OutputPortMessageModes=m  NumberInputPorts=4
      settings: InputPortMap=u1,u2,u3,u4
  Queue_ECR : Queue  InputPortMessageModes=m  OutputPortMessageModes=m
  Queue_GEM : Queue  InputPortMessageModes=m  OutputPortMessageModes=n,m  NumberEntitiesInBlock=on
      settings: OutputPortMap=o1,o5
  Queue_IT : Queue  InputPortMessageModes=m  OutputPortMessageModes=m
  Queue_PAM : Queue  InputPortMessageModes=m  OutputPortMessageModes=m
  Queue_sortie_ECR : Queue  InputPortMessageModes=m  OutputPortMessageModes=m
  Queue_sortie_GEM : Queue  InputPortMessageModes=m  OutputPortMessageModes=m
  Queue_sortie_IT : Queue  InputPortMessageModes=m  OutputPortMessageModes=m
  Queue_sortie_PAM : Queue  InputPortMessageModes=m  OutputPortMessageModes=m
  Server_ECR : EntityServer  InputPortMessageModes=m  OutputPortMessageModes=m  Capacity=1  ServiceTimeSource=Attribute  ServiceTimeAttributeName=tps_service  EntryAction=|
      | % Paramètres par catégorie [GEM, PAM, ECR, IT]
      | tau_capt = [0.94, 0.91, 0.88, 0.89];
      | debit_h  = [4.0,  3.0,  2.0,  2.0];   % t/h par ligne
      | 
      | cat = entity.categorie;
      | 
      | % Temps de service = masse / débit de la ligne [h]
      | entity.tps_service = entity.masse / debit_h(cat);
      | 
      | % Décision valorisable selon taux de captation
      | if rand() <= tau_capt(cat)
      |     entity.valorisable = 1;  % port 1 → valorisé
      | else
      |     entity.valorisable = 2;  % port 2 → refus
      | end
      | % Énergie tri optique + convoyeur tri
      | energie_spec_tri = 5.0;   % kWh/tonne
      | entity.energie_tri = entity.masse * 1000 * energie_spec_tri / 1000;
  Server_GEM : EntityServer  InputPortMessageModes=m  OutputPortMessageModes=m  Capacity=1  ServiceTimeSource=Attribute  ServiceTimeAttributeName=tps_service  EntryAction=|
      | % Paramètres par catégorie [GEM, PAM, ECR, IT]
      | tau_capt = [0.94, 0.91, 0.88, 0.89];
      | debit_h  = [4.0,  3.0,  2.0,  2.0];   % t/h par ligne
      | 
      | cat = entity.categorie;
      | 
      | % Temps de service = masse / débit de la ligne [h]
      | entity.tps_service = entity.masse / debit_h(cat);
      | 
      | % Décision valorisable selon taux de captation
      | if rand() <= tau_capt(cat)
      |     entity.valorisable = 1;  % port 1 → valorisé
      | else
      |     entity.valorisable = 2;  % port 2 → refus
      | end
      | % Énergie tri optique + convoyeur tri
      | energie_spec_tri = 5.0;   % kWh/tonne
      | entity.energie_tri = entity.masse * 1000 * energie_spec_tri / 1000;
  Server_IT : EntityServer  InputPortMessageModes=m  OutputPortMessageModes=m  Capacity=1  ServiceTimeSource=Attribute  ServiceTimeAttributeName=tps_service  EntryAction=|
      | % Paramètres par catégorie [GEM, PAM, ECR, IT]
      | tau_capt = [0.94, 0.91, 0.88, 0.89];
      | debit_h  = [4.0,  3.0,  2.0,  2.0];   % t/h par ligne
      | 
      | cat = entity.categorie;
      | 
      | % Temps de service = masse / débit de la ligne [h]
      | entity.tps_service = entity.masse / debit_h(cat);
      | 
      | % Décision valorisable selon taux de captation
      | if rand() <= tau_capt(cat)
      |     entity.valorisable = 1;  % port 1 → valorisé
      | else
      |     entity.valorisable = 2;  % port 2 → refus
      | end
      | % Énergie tri optique + convoyeur tri
      | energie_spec_tri = 5.0;   % kWh/tonne
      | entity.energie_tri = entity.masse * 1000 * energie_spec_tri / 1000;
  Server_PAM : EntityServer  InputPortMessageModes=m  OutputPortMessageModes=m  Capacity=1  ServiceTimeSource=Attribute  ServiceTimeAttributeName=tps_service  EntryAction=|
      | % Paramètres par catégorie [GEM, PAM, ECR, IT]
      | tau_capt = [0.94, 0.91, 0.88, 0.89];
      | debit_h  = [4.0,  3.0,  2.0,  2.0];   % t/h par ligne
      | 
      | cat = entity.categorie;
      | 
      | % Temps de service = masse / débit de la ligne [h]
      | entity.tps_service = entity.masse / debit_h(cat);
      | 
      | % Décision valorisable selon taux de captation
      | if rand() <= tau_capt(cat)
      |     entity.valorisable = 1;  % port 1 → valorisé
      | else
      |     entity.valorisable = 2;  % port 2 → refus
      | end
      | % Énergie tri optique + convoyeur tri
      | energie_spec_tri = 5.0;   % kWh/tonne
      | entity.energie_tri = entity.masse * 1000 * energie_spec_tri / 1000;
  Switch_ECR : EntityOutputSwitch  InputPortMessageModes=m  OutputPortMessageModes=m,m  SwitchingCriterion=From attribute  SwitchAttributeName=valorisable
  Switch_GEM : EntityOutputSwitch  InputPortMessageModes=m  OutputPortMessageModes=m,m  SwitchingCriterion=From attribute  SwitchAttributeName=valorisable
  Switch_IT : EntityOutputSwitch  InputPortMessageModes=m  OutputPortMessageModes=m,m  SwitchingCriterion=From attribute  SwitchAttributeName=valorisable
  Switch_PAM : EntityOutputSwitch  InputPortMessageModes=m  OutputPortMessageModes=m,m  SwitchingCriterion=From attribute  SwitchAttributeName=valorisable
  Out_Valorisable : Outport
  Out_Refus : Outport  Port=2
  wires:
  Entity Output Switch/1 -> Queue_GEM/1
  Queue_PAM/1 -> Server_PAM/1
  Entity Output Switch/3 -> Queue_ECR/1
  Queue_ECR/1 -> Server_ECR/1
  Entity Output Switch/4 -> Queue_IT/1
  Queue_IT/1 -> Server_IT/1
  Server_IT/1 -> Queue_sortie_IT/1
  Server_ECR/1 -> Queue_sortie_ECR/1
  Server_PAM/1 -> Queue_sortie_PAM/1
  Server_GEM/1 -> Queue_sortie_GEM/1
  Queue_sortie_PAM/1 -> Switch_PAM/1
  Queue_sortie_ECR/1 -> Switch_ECR/1
  Queue_sortie_IT/1 -> Switch_IT/1
  Queue_sortie_GEM/1 -> Switch_GEM/1
  Switch_GEM/1 -> Merge_Valorise/1
  Switch_PAM/1 -> Merge_Valorise/2
  Switch_ECR/1 -> Merge_Valorise/3
  Switch_IT/1 -> Merge_Valorise/4
  Switch_GEM/2 -> Merge_Refus/1
  Switch_PAM/2 -> Merge_Refus/2
  Switch_ECR/2 -> Merge_Refus/3
  Switch_IT/2 -> Merge_Refus/4
  Merge_Refus/1 -> Out_Refus/1
  Merge_Valorise/1 -> Out_Valorisable/1
  Entity Output Switch/2 -> Queue_PAM/1
  Queue_GEM/2 -> Server_GEM/1
  Queue_GEM/1 -> Display/1
  In_Sain/1 -> Entity Output Switch/1
